simulink model "legTra"  (R2023b)
settings: Solver=daessc  StartTime=0.0  StopTime=0.5  RelTol=1e-3
values from neighbouring files (symbols this model uses):
  X = linspace(0,3*pi/4,100)    [trajectory.m]
undefined symbols (not defined in the file or in its folder): Y, Z
libraries: sm_lib x15, nesl_utility x10
settings Model: Creator=a123  LastModifiedBy=a123

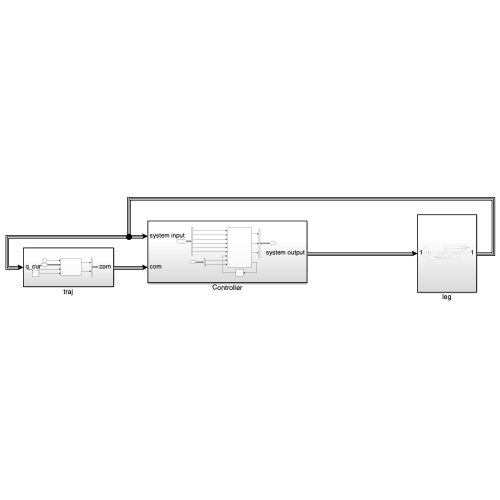
[thumbnail: Simulink's stored preview of the top-level diagram]
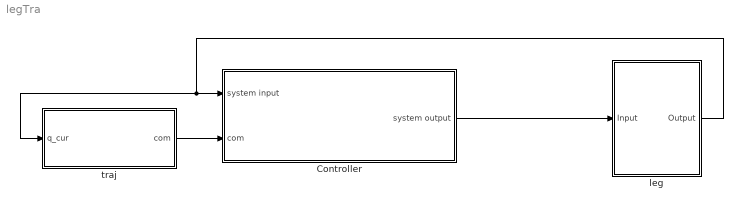
== system legTra ==
  Controller : Subsystem
  leg : Subsystem
  traj : Subsystem
  wires:
  Controller/1(system output) -> leg/1(Input)
  leg/1(Output) -> traj/1(q_cur), Controller/1(system input)
  traj/1(com) -> Controller/2(com)

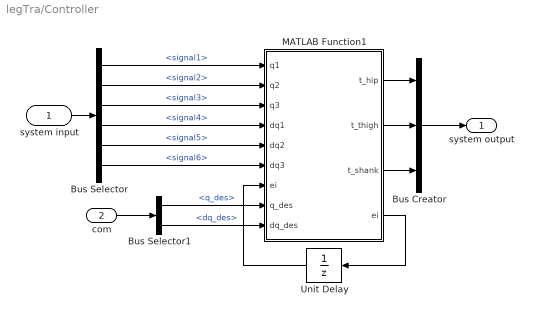
== system legTra/Controller ==
  system input : Inport
  com : Inport  Port=2
  Bus Creator : BusCreator  Inputs=3
  Bus Selector : BusSelector  OutputSignals=signal1,signal2,signal3,signal4,signal5,signal6
  Bus Selector1 : BusSelector  OutputSignals=q_des,dq_des
  MATLAB Function1 : MATLAB Function  TreatAsAtomicUnit=on
  Unit Delay : UnitDelay  InitialCondition=[0 0 0]  SampleTime=-1  HasFrameUpgradeWarning=on
  system output : Outport
  wires:
  Bus Creator/1 -> system output/1
  system input/1 -> Bus Selector/1
  Bus Selector/1 -> MATLAB Function1/1(q1)  "<signal1>"
  Bus Selector/2 -> MATLAB Function1/2(q2)  "<signal2>"
  Bus Selector/3 -> MATLAB Function1/3(q3)  "<signal3>"
  Bus Selector/4 -> MATLAB Function1/4(dq1)  "<signal4>"
  Bus Selector/5 -> MATLAB Function1/5(dq2)  "<signal5>"
  Bus Selector/6 -> MATLAB Function1/6(dq3)  "<signal6>"
  MATLAB Function1/1(t_hip) -> Bus Creator/1
  MATLAB Function1/2(t_thigh) -> Bus Creator/2
  MATLAB Function1/3(t_shank) -> Bus Creator/3
  MATLAB Function1/4(ei) -> Unit Delay/1
  Unit Delay/1 -> MATLAB Function1/7("ei ")
  Bus Selector1/1 -> MATLAB Function1/8(q_des)  "<q_des>"
  com/1 -> Bus Selector1/1
  Bus Selector1/2 -> MATLAB Function1/9(dq_des)  "<dq_des>"

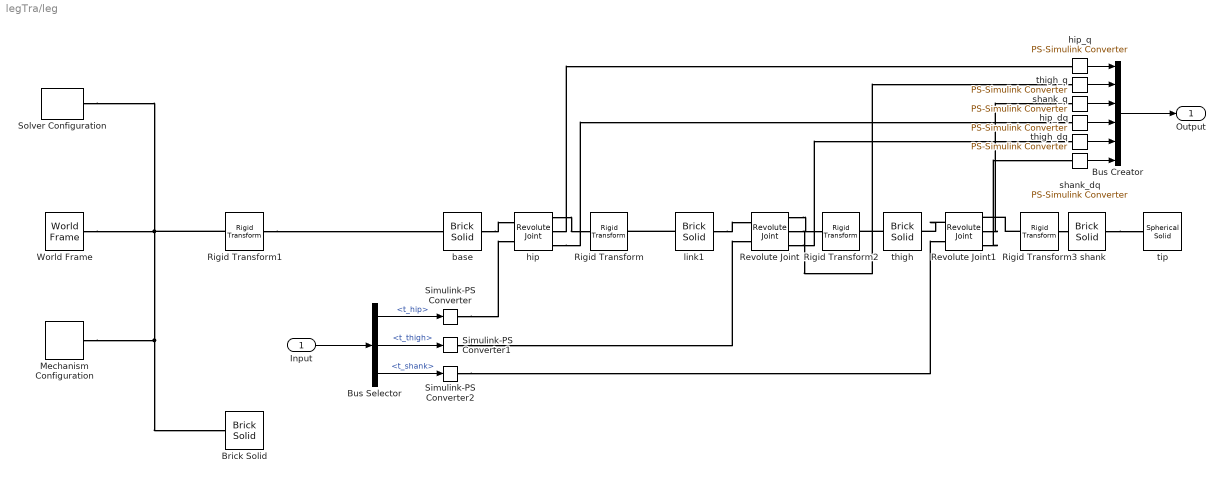
== system legTra/leg ==
  Input : Inport
  Brick Solid : sm_lib/Body Elements/Brick Solid  GraphicAmbientColor=[0.15 0.15 0.15 1.0]  BasedOnType=Density  BrickDimensions=[5 0.01 5]  BrickDimensionsUnits=m  CenterOfMass=[0 0 0]  CenterOfMassUnits=m  GraphicDiffuseColor=[0.5 0.5 0.5]  Density=1000  DensityUnits=kg/m^3  DoExposeReferenceFrame=on  GraphicEmissiveColor=[0.0 0.0 0.0 1.0]  ExportEntireGeometry=off  SerializedFrames=<Frames/>  MarkerShape=Sphere  MarkerSize=10  GraphicType=FromGeometry  InertiaType=CalculateFromGeometry  Mass=1  MassUnits=kg  MomentsOfInertia=[1 1 1]  MomentsOfInertiaUnits=kg*m^2  GraphicOpacity=1.0  ProductsOfInertia=[0 0 0]  ProductsOfInertiaUnits=kg*m^2  GraphicShininess=75  GraphicSpecularColor=[0.5 0.5 0.5 1.0]  GraphicVisPropType=SimpleVisualProperties
  Bus Creator : BusCreator  Inputs=6
  Bus Selector : BusSelector  OutputSignals=t_hip,t_thigh,t_shank
  Mechanism Configuration : sm_lib/Utilities/Mechanism Configuration  UniformGravity=Constant  GravityVector=[0 -9.80665 0]  GravityVectorUnits=m/s^2  LinearizationDelta=0.001  JointModeTransitionNonlinearIterations=2
  Revolute Joint : sm_lib/Joints/Revolute Joint  JointMode=Normal  SenseConstraintForce=off  SenseConstraintForceX=off  SenseConstraintForceY=off  SenseConstraintForceZ=off  SenseConstraintTorque=off  SenseConstraintTorqueX=off  SenseConstraintTorqueY=off  SenseConstraintTorqueZ=off  SenseTotalForce=off  SenseTotalForceX=off  SenseTotalForceY=off  SenseTotalForceZ=off  SenseTotalTorque=off  SenseTotalTorqueX=off  SenseTotalTorqueY=off  SenseTotalTorqueZ=off  CompositeWrenchDir=FollowerOnBase  CompositeWrenchFrame=BaseFrame  EquilibriumPosition=0  EquilibriumPositionUnits=deg  SpringStiffness=0  SpringStiffnessUnits=N*m/deg  DampingCoefficient=0  DampingCoefficientUnits=N*m/(deg/s)  TorqueActuationMode=InputTorque  MotionActuationMode=ComputedMotion  SensePosition=on  SenseVelocity=on  SenseAcceleration=off  SenseTorqueForce=off  SenseLowerLimitTorqueForce=off  SenseUpperLimitTorqueForce=off  LowerLimitSpecify=off  LowerLimitBound=-90  LowerLimitBoundUnits=deg  LowerLimitStiffness=1e4  LowerLimitStiffnessUnits=N*m/deg  LowerLimitDamping=10  LowerLimitDampingUnits=N*m/(deg/s)  LowerLimitTransitionRegionWidth=0.1  LowerLimitTransitionRegionWidthUnits=deg  UpperLimitSpecify=off  UpperLimitBound=90  UpperLimitBoundUnits=deg  UpperLimitStiffness=1e4  UpperLimitStiffnessUnits=N*m/deg  UpperLimitDamping=10  UpperLimitDampingUnits=N*m/(deg/s)  UpperLimitTransitionRegionWidth=0.1  UpperLimitTransitionRegionWidthUnits=deg  PositionTargetSpecify=on  PositionTargetPriority=High  PositionTargetValue=-60  PositionTargetValueUnits=deg  VelocityTargetSpecify=off  VelocityTargetPriority=High  VelocityTargetValue=0  VelocityTargetValueUnits=deg/s
  Revolute Joint1 : sm_lib/Joints/Revolute Joint  JointMode=Normal  SenseConstraintForce=off  SenseConstraintForceX=off  SenseConstraintForceY=off  SenseConstraintForceZ=off  SenseConstraintTorque=off  SenseConstraintTorqueX=off  SenseConstraintTorqueY=off  SenseConstraintTorqueZ=off  SenseTotalForce=off  SenseTotalForceX=off  SenseTotalForceY=off  SenseTotalForceZ=off  SenseTotalTorque=off  SenseTotalTorqueX=off  SenseTotalTorqueY=off  SenseTotalTorqueZ=off  CompositeWrenchDir=FollowerOnBase  CompositeWrenchFrame=BaseFrame  EquilibriumPosition=0  EquilibriumPositionUnits=deg  SpringStiffness=0  SpringStiffnessUnits=N*m/deg  DampingCoefficient=0  DampingCoefficientUnits=N*m/(deg/s)  TorqueActuationMode=InputTorque  MotionActuationMode=ComputedMotion  SensePosition=on  SenseVelocity=on  SenseAcceleration=off  SenseTorqueForce=off  SenseLowerLimitTorqueForce=off  SenseUpperLimitTorqueForce=off  LowerLimitSpecify=off  LowerLimitBound=-90  LowerLimitBoundUnits=deg  LowerLimitStiffness=1e4  LowerLimitStiffnessUnits=N*m/deg  LowerLimitDamping=10  LowerLimitDampingUnits=N*m/(deg/s)  LowerLimitTransitionRegionWidth=0.1  LowerLimitTransitionRegionWidthUnits=deg  UpperLimitSpecify=off  UpperLimitBound=90  UpperLimitBoundUnits=deg  UpperLimitStiffness=1e4  UpperLimitStiffnessUnits=N*m/deg  UpperLimitDamping=10  UpperLimitDampingUnits=N*m/(deg/s)  UpperLimitTransitionRegionWidth=0.1  UpperLimitTransitionRegionWidthUnits=deg  PositionTargetSpecify=on  PositionTargetPriority=Low  PositionTargetValue=120  PositionTargetValueUnits=deg  VelocityTargetSpecify=off  VelocityTargetPriority=High  VelocityTargetValue=0  VelocityTargetValueUnits=deg/s
  Rigid Transform : sm_lib/Frames and Transforms/Rigid Transform  TranslationMethod=Cartesian  TranslationStandardOffset=0  TranslationStandardOffsetUnits=m  TranslationStandardAxis=+Z  TranslationCartesianOffset=[0.1 0 0]  TranslationCartesianOffsetUnits=m  TranslationROffset=0  TranslationROffsetUnits=m  TranslationZOffset=0  TranslationZOffsetUnits=m  TranslationThetaOffset=0  TranslationThetaOffsetUnits=deg  RotationMethod=None  RotationAngleUnits=deg  RotationStandardAxis=+Z  RotationAngle=0.0  RotationArbitraryAxis=[0 0 1]  FollAlignAxisA=+X  BaseAlignAxisA=+Y  FollAlignAxisB=+Y  BaseAlignAxisB=+Z  RotationSequenceAxes=FollowerAxes  RotationSequence=XYX  RotationSequenceAngles=[0 0 0]  RotationSequenceAnglesUnits=deg  RotationMatrix=[1 0 0; 0 1 0; 0 0 1]  Quaternion=[1 0 0 0]
  Rigid Transform1 : sm_lib/Frames and Transforms/Rigid Transform  TranslationMethod=Cartesian  TranslationStandardOffset=0  TranslationStandardOffsetUnits=m  TranslationStandardAxis=+Z  TranslationCartesianOffset=[0 3 0]  TranslationCartesianOffsetUnits=m  TranslationROffset=0  TranslationROffsetUnits=m  TranslationZOffset=0  TranslationZOffsetUnits=m  TranslationThetaOffset=0  TranslationThetaOffsetUnits=deg  RotationMethod=None  RotationAngleUnits=deg  RotationStandardAxis=+Z  RotationAngle=0.0  RotationArbitraryAxis=[0 0 1]  FollAlignAxisA=+X  BaseAlignAxisA=+Y  FollAlignAxisB=+Y  BaseAlignAxisB=+Z  RotationSequenceAxes=FollowerAxes  RotationSequence=XYX  RotationSequenceAngles=[0 0 0]  RotationSequenceAnglesUnits=deg  RotationMatrix=[1 0 0; 0 1 0; 0 0 1]  Quaternion=[1 0 0 0]
  Rigid Transform2 : sm_lib/Frames and Transforms/Rigid Transform  TranslationMethod=Cartesian  TranslationStandardOffset=0  TranslationStandardOffsetUnits=m  TranslationStandardAxis=+Z  TranslationCartesianOffset=[0 -0.4 0]  TranslationCartesianOffsetUnits=m  TranslationROffset=0  TranslationROffsetUnits=m  TranslationZOffset=0  TranslationZOffsetUnits=m  TranslationThetaOffset=0  TranslationThetaOffsetUnits=deg  RotationMethod=None  RotationAngleUnits=deg  RotationStandardAxis=+Z  RotationAngle=0.0  RotationArbitraryAxis=[0 0 1]  FollAlignAxisA=+X  BaseAlignAxisA=+Y  FollAlignAxisB=+Y  BaseAlignAxisB=+Z  RotationSequenceAxes=FollowerAxes  RotationSequence=XYX  RotationSequenceAngles=[0 0 0]  RotationSequenceAnglesUnits=deg  RotationMatrix=[1 0 0; 0 1 0; 0 0 1]  Quaternion=[1 0 0 0]
  Rigid Transform3 : sm_lib/Frames and Transforms/Rigid Transform  TranslationMethod=Cartesian  TranslationStandardOffset=0  TranslationStandardOffsetUnits=m  TranslationStandardAxis=+Z  TranslationCartesianOffset=[0 -0.4 0]  TranslationCartesianOffsetUnits=m  TranslationROffset=0  TranslationROffsetUnits=m  TranslationZOffset=0  TranslationZOffsetUnits=m  TranslationThetaOffset=0  TranslationThetaOffsetUnits=deg  RotationMethod=None  RotationAngleUnits=deg  RotationStandardAxis=+Z  RotationAngle=0.0  RotationArbitraryAxis=[0 0 1]  FollAlignAxisA=+X  BaseAlignAxisA=+Y  FollAlignAxisB=+Y  BaseAlignAxisB=+Z  RotationSequenceAxes=FollowerAxes  RotationSequence=XYX  RotationSequenceAngles=[0 0 0]  RotationSequenceAnglesUnits=deg  RotationMatrix=[1 0 0; 0 1 0; 0 0 1]  Quaternion=[1 0 0 0]
  Simulink-PS Converter : nesl_utility/Simulink-PS Converter  PhysicalDomain=network_engine_domain  SubClassName=ps_input  LeftPortType=input  RightPortType=output  PseudoPeriodic=off  Frequencies=[]  NoiseDistribution=none  NoiseParameters=[]  Unit=1  AffineConversion=off  FilteringAndDerivatives=provide  SimscapeFilterOrder=1  InputFilterTimeConstant=0.001  UdotUserProvided=0
  Simulink-PS Converter1 : nesl_utility/Simulink-PS Converter  PhysicalDomain=network_engine_domain  SubClassName=ps_input  LeftPortType=input  RightPortType=output  PseudoPeriodic=off  Frequencies=[]  NoiseDistribution=none  NoiseParameters=[]  Unit=1  AffineConversion=off  FilteringAndDerivatives=provide  SimscapeFilterOrder=1  InputFilterTimeConstant=0.001  UdotUserProvided=0
  Simulink-PS Converter2 : nesl_utility/Simulink-PS Converter  PhysicalDomain=network_engine_domain  SubClassName=ps_input  LeftPortType=input  RightPortType=output  PseudoPeriodic=off  Frequencies=[]  NoiseDistribution=none  NoiseParameters=[]  Unit=1  AffineConversion=off  FilteringAndDerivatives=provide  SimscapeFilterOrder=1  InputFilterTimeConstant=0.001  UdotUserProvided=0
  Solver Configuration : nesl_utility/Solver Configuration  PhysicalDomain=network_engine_domain  SubClassName=solver  LeftPortType=input  RightPortType=generic  Tones=[]  Harmonics=[]  SimulateNoise=off  Profile=off  UseLocalSampling=off  EnableSwitchedLinearOptims=on  FrequencyDomain=off  UseCCode=off  RelTol=0.001  AbsTol=0.001  MinStep=1e-09  ToWorkspace=off  RevertToSquareIcSolve=off  NumHomotopyIterations=100  PhasorMode=off  PhasorModeNumHarmonics=1  ConsistencySolver=NEWTON_XTOL_AFTER_FTOL  IndexReductionMethod=DerivativeReplacement  DoDC=off  ResidualTolerance=1e-09  ConsistencyTolSource=GLOBAL  ConsistencyAbsTol=0.001  ConsistencyRelTol=0.001  ConsistencyTolFactor=0.001  UseLocalSolver=off  LocalSolverChoice=NE_BACKWARD_EULER_ADVANCER  ResolveIndetEquations=on  FunctionEvalNumThread=1  LocalSolverSampleTime=0.001  DoFixedCost=off  MaxNonlinIter=3  MaxModeIter=2  ComputeImpulses=off  ImpulseIterations=2  LinearAlgebra=auto  LinearAlgebraNumThread=0  EquationFormulation=NE_TIME_EF  DelaysMemoryBudget=1024  AutomaticFiltering=on  FilteringTimeConstant=0.001  PartitionStorageMethod=AS_NEEDED  PartitionMemoryBudget=1024  PartitionMethod=ROBUST  MultibodyUseLocalSolver=off  MultibodyLocalSolverChoice=ODE1  MultibodyLocalSolverSampleTime=0.001
  World Frame : sm_lib/Frames and Transforms/World Frame
  base : sm_lib/Body Elements/Brick Solid  GraphicAmbientColor=[0.15 0.15 0.15 1.0]  BasedOnType=Density  BrickDimensions=[0.05 0.05 0.05]  BrickDimensionsUnits=m  CenterOfMass=[0 0 0]  CenterOfMassUnits=m  GraphicDiffuseColor=[0.0 0.8 0.8]  Density=1000  DensityUnits=kg/m^3  DoExposeReferenceFrame=on  GraphicEmissiveColor=[0.0 0.0 0.0 1.0]  ExportEntireGeometry=off  SerializedFrames=<Frames><Frame><Id>Frame1</Id><Value><Name>hip</Name><Origin><Source>GeometricFeature</Source><FeatureName>+z surface</FeatureName></Origin><PrimaryAxis><DefinedDirection>+Z</DefinedDirection><Source>ReferenceFrame</Source><SourceDirection>-X</SourceDirection><FeatureName></FeatureName></PrimaryAxis><SecondaryAxis><DefinedDirection>+X</DefinedDirection><Source>ReferenceFrame</Source><SourceDirection>+Z</SourceDirection><FeatureName></FeatureName></SecondaryAxis></Value></Frame></Frames>  MarkerShape=Sphere  MarkerSize=10  GraphicType=FromGeometry  InertiaType=CalculateFromGeometry  Mass=1  MassUnits=kg  MomentsOfInertia=[1 1 1]  MomentsOfInertiaUnits=kg*m^2  GraphicOpacity=1.0  ProductsOfInertia=[0 0 0]  ProductsOfInertiaUnits=kg*m^2  GraphicShininess=75  GraphicSpecularColor=[0.5 0.5 0.5 1.0]  GraphicVisPropType=SimpleVisualProperties
  hip : sm_lib/Joints/Revolute Joint  JointMode=Normal  SenseConstraintForce=off  SenseConstraintForceX=off  SenseConstraintForceY=off  SenseConstraintForceZ=off  SenseConstraintTorque=off  SenseConstraintTorqueX=off  SenseConstraintTorqueY=off  SenseConstraintTorqueZ=off  SenseTotalForce=off  SenseTotalForceX=off  SenseTotalForceY=off  SenseTotalForceZ=off  SenseTotalTorque=off  SenseTotalTorqueX=off  SenseTotalTorqueY=off  SenseTotalTorqueZ=off  CompositeWrenchDir=FollowerOnBase  CompositeWrenchFrame=BaseFrame  EquilibriumPosition=0  EquilibriumPositionUnits=deg  SpringStiffness=0  SpringStiffnessUnits=N*m/deg  DampingCoefficient=0  DampingCoefficientUnits=N*m/(deg/s)  TorqueActuationMode=InputTorque  MotionActuationMode=ComputedMotion  SensePosition=on  SenseVelocity=on  SenseAcceleration=off  SenseTorqueForce=off  SenseLowerLimitTorqueForce=off  SenseUpperLimitTorqueForce=off  LowerLimitSpecify=off  LowerLimitBound=-90  LowerLimitBoundUnits=deg  LowerLimitStiffness=1e4  LowerLimitStiffnessUnits=N*m/deg  LowerLimitDamping=10  LowerLimitDampingUnits=N*m/(deg/s)  LowerLimitTransitionRegionWidth=0.1  LowerLimitTransitionRegionWidthUnits=deg  UpperLimitSpecify=off  UpperLimitBound=90  UpperLimitBoundUnits=deg  UpperLimitStiffness=1e4  UpperLimitStiffnessUnits=N*m/deg  UpperLimitDamping=10  UpperLimitDampingUnits=N*m/(deg/s)  UpperLimitTransitionRegionWidth=0.1  UpperLimitTransitionRegionWidthUnits=deg  PositionTargetSpecify=off  PositionTargetPriority=High  PositionTargetValue=0  PositionTargetValueUnits=deg  VelocityTargetSpecify=off  VelocityTargetPriority=High  VelocityTargetValue=0  VelocityTargetValueUnits=deg/s
  hip_dq : nesl_utility/PS-Simulink Converter  PhysicalDomain=network_engine_domain  SubClassName=ps_output  LeftPortType=input  RightPortType=output  PseudoPeriodic=off  Frequencies=[]  VectorFormat=inherit  Unit=inherit  AffineConversion=off
  hip_q : nesl_utility/PS-Simulink Converter  PhysicalDomain=network_engine_domain  SubClassName=ps_output  LeftPortType=input  RightPortType=output  PseudoPeriodic=off  Frequencies=[]  VectorFormat=inherit  Unit=inherit  AffineConversion=off
  link1 : sm_lib/Body Elements/Brick Solid  GraphicAmbientColor=[0.15 0.15 0.15 1.0]  BasedOnType=Mass  BrickDimensions=[0.2 0.05 0.05]  BrickDimensionsUnits=m  CenterOfMass=[0 0 0]  CenterOfMassUnits=m  GraphicDiffuseColor=[0.5 0.5 0.5]  Density=1000  DensityUnits=kg/m^3  DoExposeReferenceFrame=on  GraphicEmissiveColor=[0.0 0.0 0.0 1.0]  ExportEntireGeometry=off  SerializedFrames=<Frames><Frame><Id>Frame1</Id><Value><Name>thigh</Name><Origin><Source>GeometricFeature</Source><FeatureName>+x surface</FeatureName></Origin><PrimaryAxis><DefinedDirection>+Z</DefinedDirection><Source>ReferenceFrame</Source><SourceDirection>+X</SourceDirection><FeatureName></FeatureName></PrimaryAxis><SecondaryAxis><DefinedDirection>+X</DefinedDirection><Source>ReferenceFrame</Source><SourceDirection>-Z</SourceDirection><FeatureName></FeatureName></SecondaryAxis></Value></Frame></Frames>  MarkerShape=Sphere  MarkerSize=10  GraphicType=FromGeometry  InertiaType=CalculateFromGeometry  Mass=0.2  MassUnits=kg  MomentsOfInertia=[1 1 1]  MomentsOfInertiaUnits=kg*m^2  GraphicOpacity=1.0  ProductsOfInertia=[0 0 0]  ProductsOfInertiaUnits=kg*m^2  GraphicShininess=75  GraphicSpecularColor=[0.5 0.5 0.5 1.0]  GraphicVisPropType=SimpleVisualProperties
  shank : sm_lib/Body Elements/Brick Solid  GraphicAmbientColor=[0.15 0.15 0.15 1.0]  BasedOnType=Mass  BrickDimensions=[0.07 0.8 0.07]  BrickDimensionsUnits=m  CenterOfMass=[0 0 0]  CenterOfMassUnits=m  GraphicDiffuseColor=[0.5 0.5 0.5]  Density=1000  DensityUnits=kg/m^3  DoExposeReferenceFrame=on  GraphicEmissiveColor=[0.0 0.0 0.0 1.0]  ExportEntireGeometry=off  SerializedFrames=<Frames><Frame><Id>Frame1</Id><Value><Name>F1</Name><Origin><Source>GeometricFeature</Source><FeatureName>-y surface</FeatureName></Origin><PrimaryAxis><DefinedDirection>+Z</DefinedDirection><Source>ReferenceFrame</Source><SourceDirection>+Z</SourceDirection><FeatureName></FeatureName></PrimaryAxis><SecondaryAxis><DefinedDirection>+X</DefinedDirection><Source>ReferenceFrame</Source><SourceDirection>+X</SourceDirection><FeatureName></FeatureName></SecondaryAxis></Value></Frame></Frames>  MarkerShape=Sphere  MarkerSize=10  GraphicType=FromGeometry  InertiaType=CalculateFromGeometry  Mass=0.5  MassUnits=kg  MomentsOfInertia=[1 1 1]  MomentsOfInertiaUnits=kg*m^2  GraphicOpacity=1.0  ProductsOfInertia=[0 0 0]  ProductsOfInertiaUnits=kg*m^2  GraphicShininess=75  GraphicSpecularColor=[0.5 0.5 0.5 1.0]  GraphicVisPropType=SimpleVisualProperties
  shank_dq : nesl_utility/PS-Simulink Converter  PhysicalDomain=network_engine_domain  SubClassName=ps_output  LeftPortType=input  RightPortType=output  PseudoPeriodic=off  Frequencies=[]  VectorFormat=inherit  Unit=inherit  AffineConversion=off
  shank_q : nesl_utility/PS-Simulink Converter  PhysicalDomain=network_engine_domain  SubClassName=ps_output  LeftPortType=input  RightPortType=output  PseudoPeriodic=off  Frequencies=[]  VectorFormat=inherit  Unit=inherit  AffineConversion=off
  thigh : sm_lib/Body Elements/Brick Solid  GraphicAmbientColor=[0.15 0.15 0.15 1.0]  BasedOnType=Mass  BrickDimensions=[0.07 0.8 0.07]  BrickDimensionsUnits=m  CenterOfMass=[0 0 0]  CenterOfMassUnits=m  GraphicDiffuseColor=[0.5 0.5 0.5]  Density=1000  DensityUnits=kg/m^3  DoExposeReferenceFrame=on  GraphicEmissiveColor=[0.0 0.0 0.0 1.0]  ExportEntireGeometry=off  SerializedFrames=<Frames><Frame><Id>Frame1</Id><Value><Name>F1</Name><Origin><Source>GeometricFeature</Source><FeatureName>-y surface</FeatureName></Origin><PrimaryAxis><DefinedDirection>+Z</DefinedDirection><Source>ReferenceFrame</Source><SourceDirection>+Z</SourceDirection><FeatureName></FeatureName></PrimaryAxis><SecondaryAxis><DefinedDirection>+Y</DefinedDirection><Source>ReferenceFrame</Source><SourceDirection>+Y</SourceDirection><FeatureName></FeatureName></SecondaryAxis></Value></Frame></Frames>  MarkerShape=Sphere  MarkerSize=10  GraphicType=FromGeometry  InertiaType=CalculateFromGeometry  Mass=0.5  MassUnits=kg  MomentsOfInertia=[1 1 1]  MomentsOfInertiaUnits=kg*m^2  GraphicOpacity=1.0  ProductsOfInertia=[0 0 0]  ProductsOfInertiaUnits=kg*m^2  GraphicShininess=75  GraphicSpecularColor=[0.5 0.5 0.5 1.0]  GraphicVisPropType=SimpleVisualProperties
  thigh_dq : nesl_utility/PS-Simulink Converter  PhysicalDomain=network_engine_domain  SubClassName=ps_output  LeftPortType=input  RightPortType=output  PseudoPeriodic=off  Frequencies=[]  VectorFormat=inherit  Unit=inherit  AffineConversion=off
  thigh_q : nesl_utility/PS-Simulink Converter  PhysicalDomain=network_engine_domain  SubClassName=ps_output  LeftPortType=input  RightPortType=output  PseudoPeriodic=off  Frequencies=[]  VectorFormat=inherit  Unit=inherit  AffineConversion=off
  tip : sm_lib/Body Elements/Spherical Solid  GraphicAmbientColor=[0.15 0.15 0.15 1.0]  BasedOnType=Mass  CenterOfMass=[0 0 0]  CenterOfMassUnits=m  GraphicDiffuseColor=[0.0 1.0 0.6]  Density=1000  DensityUnits=kg/m^3  DoExposeReferenceFrame=on  GraphicEmissiveColor=[0.0 0.0 0.0 1.0]  ExportEntireGeometry=off  SerializedExposedGeometries=<exposedGeometries/>  SerializedFrames=<Frames/>  MarkerShape=Sphere  MarkerSize=10  GraphicType=FromGeometry  InertiaType=CalculateFromGeometry  Mass=0.01  MassUnits=kg  MomentsOfInertia=[1 1 1]  MomentsOfInertiaUnits=kg*m^2  GraphicOpacity=1.0  ProductsOfInertia=[0 0 0]  ProductsOfInertiaUnits=kg*m^2  GraphicShininess=75  GraphicSpecularColor=[0.5 0.5 0.5 1.0]  SphereRadius=0.08  SphereRadiusUnits=m  GraphicVisPropType=SimpleVisualProperties
  Output : Outport
  wires:
  Input/1 -> Bus Selector/1
  Bus Selector/1 -> Simulink-PS Converter/1  "<t_hip>"
  hip_q/1 -> Bus Creator/1
  thigh_q/1 -> Bus Creator/2
  shank_q/1 -> Bus Creator/3
  hip_dq/1 -> Bus Creator/4
  thigh_dq/1 -> Bus Creator/5
  shank_dq/1 -> Bus Creator/6
  Bus Creator/1 -> Output/1
  Bus Selector/2 -> Simulink-PS Converter1/1  "<t_thigh>"
  Bus Selector/3 -> Simulink-PS Converter2/1  "<t_shank>"
  connections:
  Revolute Joint/RConn2 -- thigh_q/LConn1
  hip/RConn2 -- hip_q/LConn1
  base/LConn1 -- hip/LConn1
  thigh/RConn1 -- Rigid Transform2/RConn1
  link1/LConn1 -- Revolute Joint/LConn1
  Rigid Transform3/RConn1 -- shank/RConn1
  Rigid Transform3/LConn1 -- Revolute Joint1/RConn1
  hip/RConn1 -- Rigid Transform/LConn1
  Revolute Joint/RConn3 -- thigh_dq/LConn1
  Revolute Joint/RConn1 -- Rigid Transform2/LConn1
  hip/RConn3 -- hip_dq/LConn1
  link1/RConn1 -- Rigid Transform/RConn1
  Solver Configuration/RConn1 -- Mechanism Configuration/RConn1 -- Brick Solid/RConn1 -- Rigid Transform1/LConn1 -- World Frame/RConn1
  shank/LConn1 -- tip/RConn1
  Rigid Transform1/RConn1 -- base/RConn1
  Revolute Joint1/RConn3 -- shank_dq/LConn1
  Revolute Joint1/LConn1 -- thigh/LConn1
  Revolute Joint1/RConn2 -- shank_q/LConn1
  Simulink-PS Converter/RConn1 -- hip/LConn2
  Simulink-PS Converter1/RConn1 -- Revolute Joint/LConn2
  Simulink-PS Converter2/RConn1 -- Revolute Joint1/LConn2

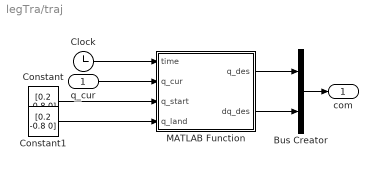
== system legTra/traj ==
  q_cur : Inport
  Bus Creator : BusCreator  Inputs=2
  Clock : Clock
  Constant : Constant  Value=[0.2 -0.8 0]
  Constant1 : Constant  Value=[0.2 -0.8 0]
  MATLAB Function : MATLAB Function  TreatAsAtomicUnit=on
  com : Outport
  wires:
  Bus Creator/1 -> com/1
  Clock/1 -> MATLAB Function/1(time)
  q_cur/1 -> MATLAB Function/2(q_cur)
  Constant/1 -> MATLAB Function/3(q_start)
  Constant1/1 -> MATLAB Function/4(q_land)
  MATLAB Function/1(q_des) -> Bus Creator/1
  MATLAB Function/2(dq_des) -> Bus Creator/2

== matlab function legTra/Controller/MATLAB Function1 ==
  data: t_hip output; t_thigh output; t_shank output; q1 input; q2 input; q3 input; dq1 input; dq2 input; dq3 input; ei input; ei output; q_des input; dq_des input
function [t_hip,t_thigh,t_shank,ei] = leg_controller(q1,q2,q3,dq1,dq2,dq3,ei,q_des,dq_des)
q_states = [q1;q2;q3];
dq_states = [dq1;dq2;dq3];

e_q = q_des - q_states;
e_dq = dq_des - dq_states;

%PID参数
% kp = [3000;350;450]; 
kp = [600;650;650];
ki = [1;1.5;0.5];
kd = [10;65;60];
tqs = kp .* e_q + kd' .* e_dq + ki .* ei; %系统PID控制器输出序列
% Ee = Ee + e_prev;       %累积偏差

t_hip = tqs(1);
t_thigh = tqs(2);
t_shank = tqs(3);
ei = ei + e_q;
end

== matlab function legTra/traj/MATLAB Function ==
  data: time input; q_des output; dq_des output; q_cur input; q_start input; q_land input
function [q_des, dq_des] = genTraj(time,q_cur,q_start,q_land)
T = 0.5;
p = time/T;
h = 0.4;

l1 = 0.2;
l2 = 0.8;
l3 = 0.8;

xl = q_land(1);
yl = q_land(2);
zl = q_land(3);

x0 = q_start(1);
y0 = q_start(2);
z0 = q_start(3);

%% 正运动学部分
t1 = q_cur(1);
t2 = q_cur(2);
t3 = q_cur(3);

% % x
% xc = l3*sin(t2 + t3) + l2*sin(t2);
% % y
% yc = l3*(cos(t1)*sin(t2)*sin(t3) - cos(t1)*cos(t2)*cos(t3)) + l1*sin(t1) - l2*cos(t1)*cos(t2);
% % z
% zc = l1*cos(t1) - l3*(sin(t1)*sin(t2)*sin(t3) - cos(t2)*cos(t3)*sin(t1)) + l2*cos(t2)*sin(t1);

%% 求解轨迹和速度
xc = x0 + (xl - x0)/(2*pi)*(2*pi*p - sin(2*pi*p));
zc = z0 + (zl - z0)/(2*pi)*(2*pi*p - sin(2*pi*p));
yc = y0 + h/2*(1 - cos(2*pi*p));

dxc = (xl - x0)/T*(1 - cos(2*pi*p));
dyc = (yl - y0)/T*(1 - cos(2*pi*p));
dzc = (pi*h)/T*sin(2*pi*p);

%% 逆运动学部分
% 角度
L = sqrt(xc^2 + yc^2 - l1^2);
t1c = atan2((yc * l1 + xc * L),(xc * l1 - yc * L));
t3c = pi - acos((l2^2 + l3^2 - (xc^2 + yc^2 + zc^2 - l1^2))/(2*l2*l3));
t2c_t = -(zc + (l3*(yc - (l1*(imag(l1*xc) + real(l1*yc) - imag(yc*(- l1^2 + xc^2 + yc^2)^(1/2)) + real(xc*(- l1^2 + xc^2 + yc^2)^(1/2))))/abs(l1*xc - yc*(- l1^2 + xc^2 + yc^2)^(1/2) + l1*yc*1i + xc*(- l1^2 + xc^2 + yc^2)^(1/2)*1i))*(1 - (l1^2 + l2^2 + l3^2 - xc^2 - yc^2 - zc^2)^2/(4*l2^2*l3^2))^(1/2))/((l2*(imag(l1*yc) - real(l1*xc) + imag(xc*(- l1^2 + xc^2 + yc^2)^(1/2)) + real(yc*(- l1^2 + xc^2 + yc^2)^(1/2))))/abs(l1*xc - yc*(- l1^2 + xc^2 + yc^2)^(1/2) + l1*yc*1i + xc*(- l1^2 + xc^2 + yc^2)^(1/2)*1i) - ((imag(l1*yc) - real(l1*xc) + imag(xc*(- l1^2 + xc^2 + yc^2)^(1/2)) + real(yc*(- l1^2 + xc^2 + yc^2)^(1/2)))*(l1^2 + l2^2 + l3^2 - xc^2 - yc^2 - zc^2))/(2*l2*abs(l1*xc - yc*(- l1^2 + xc^2 + yc^2)^(1/2) + l1*yc*1i + xc*(- l1^2 + xc^2 + yc^2)^(1/2)*1i))))/(l2 - l3*((l1^2 + l2^2 + l3^2 - xc^2 - yc^2 - zc^2)/(2*l2*l3) + (l3*((l1^2 + l2^2 + l3^2 - xc^2 - yc^2 - zc^2)^2/(4*l2^2*l3^2) - 1)*(imag(l1*yc) - real(l1*xc) + imag(xc*(- l1^2 + xc^2 + yc^2)^(1/2)) + real(yc*(- l1^2 + xc^2 + yc^2)^(1/2))))/(abs(l1*xc - yc*(- l1^2 + xc^2 + yc^2)^(1/2) + l1*yc*1i + xc*(- l1^2 + xc^2 + yc^2)^(1/2)*1i)*((l2*(imag(l1*yc) - real(l1*xc) + imag(xc*(- l1^2 + xc^2 + yc^2)^(1/2)) + real(yc*(- l1^2 + xc^2 + yc^2)^(1/2))))/abs(l1*xc - yc*(- l1^2 + xc^2 + yc^2)^(1/2) + l1*yc*1i + xc*(- l1^2 + xc^2 + yc^2)^(1/2)*1i) - ((imag(l1*yc) - real(l1*xc) + imag(xc*(- l1^2 + xc^2 + yc^2)^(1/2)) + real(yc*(- l1^2 + xc^2 + yc^2)^(1/2)))*(l1^2 + l2^2 + l3^2 - xc^2 - yc^2 - zc^2))/(2*l2*abs(l1*xc - yc*(- l1^2 + xc^2 + yc^2)^(1/2) + l1*yc*1i + xc*(- l1^2 + xc^2 + yc^2)^(1/2)*1i))))));
t2c = asin(t2c_t);

q_des = [t1c;t2c;t3c];

% 速度
J = [l2*cos(t1)*cos(t2) - l1*sin(t1) - l3*(cos(t1)*sin(t2)*sin(t3) - cos(t1)*cos(t2)*cos(t3)), - l3*(cos(t2)*sin(t1)*sin(t3) + cos(t3)*sin(t1)*sin(t2)) - l2*sin(t1)*sin(t2), -l3*(cos(t2)*sin(t1)*sin(t3) + cos(t3)*sin(t1)*sin(t2));
l1*cos(t1) - l3*(sin(t1)*sin(t2)*sin(t3) - cos(t2)*cos(t3)*sin(t1)) + l2*cos(t2)*sin(t1),   l3*(cos(t1)*cos(t2)*sin(t3) + cos(t1)*cos(t3)*sin(t2)) + l2*cos(t1)*sin(t2),  l3*(cos(t1)*cos(t2)*sin(t3) + cos(t1)*cos(t3)*sin(t2));
                                                                                       0,                                                - l3*cos(t2 + t3) - l2*cos(t2),                                        -l3*cos(t2 + t3)];
dq_des_temp = [dxc;dyc;dzc];
dq_des = J\dq_des_temp;
